simulink model "c221127_FCEV_SLMP_SQP"  (R2022b)
settings: Solver=FixedStepAuto  StartTime=0.0  StopTime=DrvCycLen  FixedStep=1  RelTol=1e-3
values from neighbouring files (symbols this model uses):
  AccThrshd = 1    [Config_c221112.m]    (also in Config_c221127.m; Config_c221218.m; Config_c230117.m; Config_c230321.m)
  AlphaRampFactor = 8    [Config_c221112.m]    (also in Config_c221127.m; Config_c221218.m; Config_c230117.m; Config_c230321.m)
  Bat_eff_chg_average = 0.969    [FCEV_original_data.mat]
  Bat_eff_dis_average = 0.9632    [FCEV_original_data.mat]
  Bat_end_of_life_percent = 20    [FCEV_original_data.mat]
  Bat_I_chg_max = -120    [FCEV_original_data.mat]
  Bat_I_dis_max = 200    [FCEV_original_data.mat]
  Bat_nom_Ic = 2.5    [FCEV_original_data.mat]
  Bat_nom_SOC = 0.35    [FCEV_original_data.mat]
  Bat_nom_temp_oC = 25    [FCEV_original_data.mat]
  Bat_num_pa = 9    [FCEV_original_data.mat]
  Bat_num_se = 97    [FCEV_original_data.mat]
  Bat_ori_C1_chg_F = [397.526659684 455.660832136 435.08783522 460.845064365 457.605812374 417.289828504 416.373906992 359.741413056 321.561704819 1109.14132554 1165.67733205 1135.97600211 ... (72 elements, 9x8)]    [FCEV_original_data.mat]
  Bat_ori_C1_dis_F = [187.121968588 287.083505726 346.448009002 395.529439835 387.517274826 389.973134196 432.856765051 486.92921923 512.158935268 425.990733989 614.68708868 771.472592368 ... (72 elements, 9x8)]    [FCEV_original_data.mat]
  Bat_ori_C2_chg_F = [8748.48589695 7773.35875681 9404.86567646 8934.73981058 8290.58671366 7592.78422269 7759.44623103 7396.59043829 6151.35152293 16187.7227039 11721.8480541 13157.8579836 ... (72 elements, 9x8)]    [FCEV_original_data.mat]
  Bat_ori_C2_dis_F = [2939.81325553 4590.73311898 5504.93546413 5887.5077374 6534.37836712 7765.46899768 10584.7751706 10372.0508438 9238.72693885 5207.86390693 7911.43744944 8879.62137571 ... (72 elements, 9x8)]    [FCEV_original_data.mat]
  Bat_ori_cap_max_Ah = 20.7    [Config_c221218.m]    (also in Config_c230117.m; Config_c230321.m; FCEV_original_data.mat)
  Bat_ori_dUdt4 = [-0.303773584906 -0.249056603774 -0.115094339623 -0.0396226415094 0.0396226415094 0.0641509433962 0.107547169811 0.111320754717 0.0415094339623 0.0547169811321 0.130188679245]    [FCEV_original_data.mat]
  Bat_ori_R0_chg_O = [0.0771669453735 0.0731809311402 0.0726556782939 0.0729965156794 0.0731758310684 0.0742031005051 0.0721266921026 0.0714211058078 0.0714186176143 0.0374124505155 0.0354566732504 0.0345430657188 ... (72 elements, 9x8)]    [FCEV_original_data.mat]
  Bat_ori_R0_dis_O = [0.0819458671157 0.0812429476608 0.0803749674507 0.0805513601722 0.0838629023857 0.0850797840015 0.0829875518672 0.0826388888889 0.0812514106148 0.0428124986417 0.0424658903711 0.0428572670451 ... (72 elements, 9x8)]    [FCEV_original_data.mat]
  Bat_ori_R1_chg_O = [0.114339870884 0.105392753268 0.104421193553 0.109821896183 0.114868279838 0.123333154908 0.129174812826 0.149917249373 0.174896487845 0.0420560161846 0.0390948352938 0.0370122837364 ... (72 elements, 9x8)]    [FCEV_original_data.mat]
  Bat_ori_R1_dis_O = [0.304806399643 0.213604089624 0.171463520004 0.151183840498 0.140630862434 0.128795299077 0.116857791733 0.112567113582 0.106368362501 0.0943235089866 0.0730697254134 0.0611414736086 ... (72 elements, 9x8)]    [FCEV_original_data.mat]
  Bat_ori_R2_chg_O = [0.134518959939 0.17565045702 0.161100627268 0.189032232545 0.205639040497 0.226170473035 0.223651875822 0.181765694192 0.212966950836 0.073628872144 0.0788540822416 0.0792414571734 ... (72 elements, 9x8)]    [FCEV_original_data.mat]
  Bat_ori_R2_dis_O = [0.354968099904 0.285293035102 0.286338708953 0.298763853987 0.248762838155 0.178586175471 0.129047399775 0.188406991173 0.174494800676 0.131839238891 0.123225430215 0.132069033134 ... (72 elements, 9x8)]    [FCEV_original_data.mat]
  Bat_ori_SOC2 = [0 0.001 0.002 0.003 0.004 0.005 0.006 0.007 0.008 0.009 0.01 0.011 ... (1001 elements, 1x1001)]    [FCEV_original_data.mat]
  Bat_ori_SOC4 = [-0.00598301069999 0.0920117618231 0.190864167279 0.289083557951 0.387343788287 0.485011843502 0.5850485992 0.678163031937 0.774810095565 0.876684636119 0.972739524626]    [FCEV_original_data.mat]
  Bat_ori_Uoc_chg_V = [2.4478 2.54923264342 2.6007 2.6383 2.66953057366 2.69636321708 2.7197 2.74042850391 2.75906114733 2.77619379074 2.792 2.80675907757 ... (1001 elements, 1x1001)]    [FCEV_original_data.mat]
  Bat_ori_Uoc_dis_V = [1.9998 2.03916768329 2.24724374236 2.39700902919 2.48767431602 2.5476 2.5882 2.6202 2.64771773167 2.6719 2.6933 2.71251566192 ... (1001 elements, 1x1001)]    [FCEV_original_data.mat]
  Bat_ori_Uoc_V = [2.2238 2.29420016335 2.42397187118 2.5176545146 2.57860244484 2.62198160854 2.65395 2.68031425195 2.7033894395 2.72404689537 2.74265 2.75963736975 ... (1001 elements, 1x1001)]    [FCEV_original_data.mat]
  Bat_power_max_kW = 50    [FCEV_original_data.mat]
  Bat_power_min_kW = 0    [FCEV_original_data.mat]
  Bat_single_capacity_nom_Ah = 2.3    [FCEV_original_data.mat]
  Bat_SOC_ini = 0.3    [Config_c22100601.m]    (also in Config_c22100701.m; FCEV_original_data.mat = 0.45)
  Bat_SOC_max = 0.9    [FCEV_original_data.mat]
  Bat_SOC_min = 0.3    [FCEV_original_data.mat]
  Bat_temp_amb_oC = 25    [FCEV_original_data.mat]
  Bat_temp_cool_oC = 25    [FCEV_original_data.mat]
  BattInitTemp = 25    [Config_c221127.m]    (also in Config_c221218.m; Config_c230117.m; Config_c230321.m)
  BattOnly = 0    [Config_c221218.m]    (also in Config_c230117.m = BattSocRightNow > BattSocLowerLimit; Config_c230321.m = double(BattSocRightNow > BattSocLowerLimit))
  BattSocInit = 0.9    [Config_c221112.m]    (also in Config_c221127.m = 0.3; Config_c221218.m = 0.3; Config_c230117.m = 0.8; Config_c230321.m = 0.8)
  BattSocLowerLimit = 0.25    [Config_c221112.m]    (also in Config_c221127.m = 0.3; Config_c221218.m = 0.3; Config_c230117.m = 0.3; Config_c230321.m = 0.3)
  BattSocRightNow = BattSocRightNow - SocDrop    [Config_c221218.m]    (also in Config_c230117.m; Config_c230321.m)
  BattSocUpperLimit = 0.9    [Config_c221112.m]    (also in Config_c221127.m = 0.8; Config_c221218.m = 0.8; Config_c230117.m = 0.8; Config_c230321.m = 0.8)
  CFWF = 0.5    [Config_c221127.m]    (also in Config_c221218.m; Config_c230117.m; Config_c230321.m)
  DCAC_eff = 0.95    [FCEV_original_data.mat]
  DCDC_ori_eff = [0.95 0.96 0.97 0.976 0.98 0.978 0.973 0.962]    [FCEV_original_data.mat]
  DCDC_ori_power_kW = [0 10 20 30 40 50 60 70]    [FCEV_original_data.mat]
  DeAccThrshd = -1    [Config_c221112.m]    (also in Config_c221127.m; Config_c221218.m; Config_c230117.m; Config_c230321.m)
  DeltaFcPwrRcm_down = 0.5    [Config_c221127.m]    (also in Config_c221218.m; Config_c230117.m; Config_c230321.m)
  DeltaFcPwrRcm_up = 2    [Config_c221127.m]    (also in Config_c221218.m = 3; Config_c230117.m = 4; Config_c230321.m = 4)
  DrvCycRange = sum(DrvCycVps(:,2))    [Config_c221112.m]    (also in Config_c221127.m; Config_c221218.m; Config_c230117.m; Config_c230321.m)
  FC_ori_eff = [0.1 0.33 0.492 0.533 0.559 0.596 0.591 0.562 0.508]    [FCEV_original_data.mat]
  FC_ori_fuel_rate_gps = [0 0.0505050505051 0.0846883468835 0.117260787992 0.149075730471 0.279642058166 0.423011844332 0.593119810202 0.820209973753]    [FCEV_original_data.mat]
  FC_ori_power_kW = [0 2 5 7.5 10 20 30 40 50]    [FCEV_original_data.mat]
  FC_power_max_kW = 50    [FCEV_original_data.mat]
  FC_power_min_kW = 0    [FCEV_original_data.mat]
  FcPwrDropCall = 6    [Config_c221127.m]    (also in Config_c221218.m; Config_c230117.m; Config_c230321.m)
  HydpriceRmb = 30    [Config_c221127.m]    (also in Config_c221218.m; Config_c230117.m; Config_c230321.m)
  m = Time_sample    [Config_c22100601.m]    (also in Config_c22100701.m)
  MC_eff_brk_average = 0.810578512397    [FCEV_original_data.mat]
  MC_eff_dri_average = 0.810578512397    [FCEV_original_data.mat]
  MC_inertia = 0.06    [FCEV_original_data.mat]
  MC_ori_eff = [0.7 0.78 0.85 0.86 0.81 0.82 0.79 0.78 0.78 0.78 0.78 0.7 ... (231 elements, 11x21)]    [FCEV_original_data.mat]
  MC_ori_power_brk_req_kW = [0 -28.3912930389 -56.7825860779 -85.1738791168 -113.565172156 -141.956465195 -170.347758234 -198.739051273 -227.130344311 -255.52163735 -283.912930389 0 ... (121 elements, 11x11)]    [FCEV_original_data.mat]
  MC_ori_power_dri_req_kW = [0 0 0 0 0 0 0 0 0 0 0 0 ... (121 elements, 11x11)]    [FCEV_original_data.mat]
  MC_ori_spd_rpm = [0 1000 2000 3000 4000 5000 6000 7000 8000 9000 10000]    [FCEV_original_data.mat]
  MC_ori_trq_brk_max_Nm = [-271.1368 -271.1368 -271.1368 -237.5159 -178.1369 -142.4824 -118.7579 -101.8119 -89.0685 -79.172 -71.1734]    [FCEV_original_data.mat]
  MC_ori_trq_brk_Nm = [-271.136848522 -244.02316367 -216.909478817 -189.795793965 -162.682109113 -135.568424261 -108.454739409 -81.3410545565 -54.2273697044 -27.1136848522 0]    [FCEV_original_data.mat]
  MC_ori_trq_dri_max_Nm = [271.1368 271.1368 271.1368 237.5159 178.1369 142.4824 118.7579 101.8119 89.0685 79.172 71.1734]    [FCEV_original_data.mat]
  MC_ori_trq_dri_Nm = [0 27.1136848522 54.2273697044 81.3410545565 108.454739409 135.568424261 162.682109113 189.795793965 216.909478817 244.02316367 271.136848522]    [FCEV_original_data.mat]
  MC_ori_trq_Nm = [-271.136848522 -244.02316367 -216.909478817 -189.795793965 -162.682109113 -135.568424261 -108.454739409 -81.3410545565 -54.2273697044 -27.1136848522 0 27.1136848522 ... (21 elements, 1x21)]    [FCEV_original_data.mat]
  MC_power_max_kW = 75    [FCEV_original_data.mat]
  MC_spd_max_rpm = 10000    [FCEV_original_data.mat]
  MC_spd_min_rpm = 0    [FCEV_original_data.mat]
  MC_spd_scale = 1    [FCEV_original_data.mat]
  MC_trq_scale = 1    [FCEV_original_data.mat]
  MC_U_min_V = 120    [FCEV_original_data.mat]
  no_FcPwrSlowDrop = 1    [Config_c230321.m]
  Placeholder = 0    [Config_c221127.m]    (also in Config_c221218.m; Config_c230117.m; Config_c230321.m)
  PredLen = 5    [Config_c221112.m]    (also in Config_c221127.m; Config_c221218.m; Config_c230117.m; Config_c230321.m)
  Road_u = 0.75    [FCEV_original_data.mat]
  SC_np = 1    [Config_c230321.m]
  SC_ns = 100    [Config_c230321.m]
  SC_rc = 1000    [Config_c230321.m]
  SLMP_LearningRate = 0.05    [Config_c221112.m]    (also in Config_c221127.m; Config_c221218.m; Config_c230117.m; Config_c230321.m)
  tDegTable = [zeros(1,3),linspace(0,0.13,47)]    [Config_c221127.m]    (also in Config_c221218.m; Config_c230117.m; Config_c230321.m)
  usd2rmb = 7.116    [Config_c22100601.m]    (also in Config_c22100701.m; Config_c221106.m = 6; Config_c221112.m = 6; Config_c221127.m = 6)
  Veh_air_density_kgpm2 = 1.2    [FCEV_original_data.mat]
  Veh_brk_front = [1 0.6 0.608 0.61 0.618 0.624 0.636 0.645 0.655]    [FCEV_original_data.mat]
  Veh_brk_z = [0.1 0.2 0.3 0.4 0.5 0.6 0.7 0.8 0.9]    [FCEV_original_data.mat]
  Veh_brk_z_max = 0.7    [FCEV_original_data.mat]
  Veh_brk_z_min = 0.1    [FCEV_original_data.mat]
  Veh_coeff_drag = 0.312    [FCEV_original_data.mat]
  Veh_coeff_roll = 0.00863    [FCEV_original_data.mat]
  Veh_final_drive_inertia = 0.1105    [FCEV_original_data.mat]
  Veh_final_drive_ratio = 3.47    [FCEV_original_data.mat]
  Veh_frontal_area_m2 = 2.06    [FCEV_original_data.mat]
  Veh_gravity_acc_ms2 = 9.81    [FCEV_original_data.mat]
  Veh_mass_cargo_kg = 113    [FCEV_original_data.mat]
  Veh_mass_curb_kg = 1157    [FCEV_original_data.mat]
  Veh_mech_eff = 0.9    [FCEV_original_data.mat]
  Veh_rotary_mass_conversion_factor = 1.05    [FCEV_original_data.mat]
  Veh_size_cg_height_m = 0.53    [FCEV_original_data.mat]
  Veh_wheel_inertia = 3.1039    [FCEV_original_data.mat]
  Veh_wheel_radius_m = 0.313    [FCEV_original_data.mat]
  Veh_wt_frac_front = 0.5    [FCEV_original_data.mat]
  VstdThrshd = 2    [Config_c221112.m]    (also in Config_c221127.m; Config_c221218.m; Config_c230117.m; Config_c230321.m)
undefined symbols (not defined in the file or in its folder): Bat_ori_temp, SC_iv, SC_nm, SC_SocTable
libraries: autolibshared x2
(part 2 of 8)

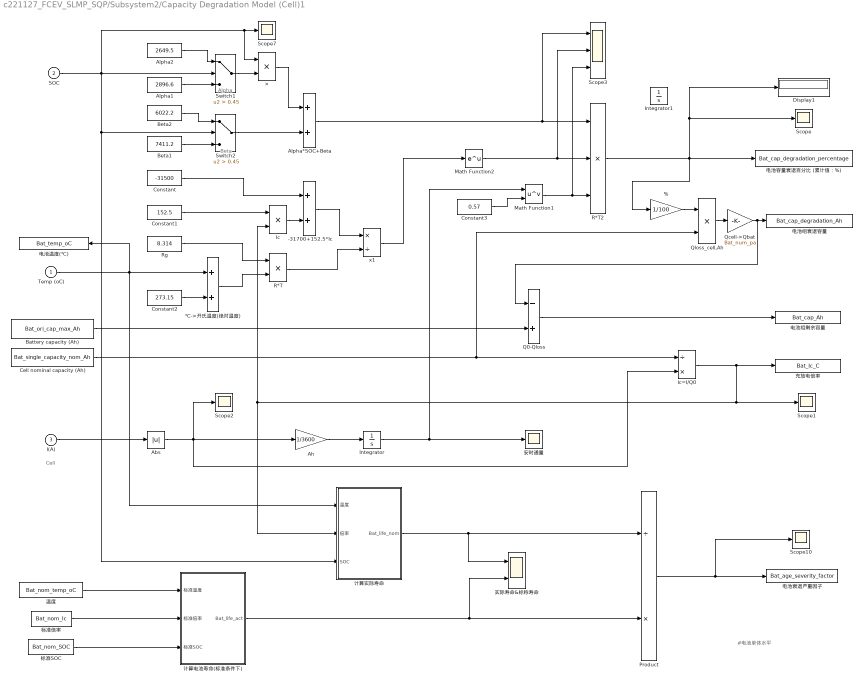
== system c221127_FCEV_SLMP_SQP/Subsystem2/Capacity Degradation Model (Cell)1 ==
  note: Cell
  note: #电池单体水平
  note: Beta
  note: Alpha
  Temp (oC) : Inport
  SOC : Inport  Port=2
  I(A) : Inport  Port=3
  % : Gain  Gain=1/100
  -31700+152.5*Ic : Sum  InputSameDT=on  SaturateOnIntegerOverflow=on  OutDataTypeStr=Inherit: Same as first input
  Abs : Abs  SaturateOnIntegerOverflow=off
  Ah : Gain  Gain=1/3600
  Alpha*SOC+Beta : Sum  InputSameDT=on  SaturateOnIntegerOverflow=on  OutDataTypeStr=Inherit: Same as first input
  Alpha1 : Constant  Value=2896.6
  Alpha2 : Constant  Value=2649.5
  Battery capacity (Ah) : Constant  Value=Bat_ori_cap_max_Ah
  Beta1 : Constant  Value=7411.2
  Beta2 : Constant  Value=6022.2
  Cell nominal capacity (Ah) : Constant  Value=Bat_single_capacity_nom_Ah
  Constant : Constant  Value=-31500
  Constant1 : Constant  Value=152.5
  Constant2 : Constant  Value=273.15
  Constant3 : Constant  Value=0.57
  Display1 : Display
  Ic : Product  InputSameDT=on  RndMeth=Zero  SaturateOnIntegerOverflow=on  OutDataTypeStr=Inherit: Same as first input
  Ic=I/Q0 : Product  Inputs=/*  InputSameDT=on  RndMeth=Zero  SaturateOnIntegerOverflow=on  OutDataTypeStr=Inherit: Same as first input
  Integrator : Integrator  InitialCondition=eps
  Integrator1 : Integrator
  Math Function1 : Math  Operator=pow  SignedPower=on
  Math Function2 : Math  SignedPower=on
  Product : Product  Inputs=/*
  Q0-Qloss : Sum  Inputs=-+  InputSameDT=on  SaturateOnIntegerOverflow=on  OutDataTypeStr=Inherit: Same as first input
  Qcell->Qbat : Gain  Gain=Bat_num_pa  SaturateOnIntegerOverflow=on  OutDataTypeStr=Inherit: Same as input  ParamDataTypeStr=Inherit: Same as input
  Qloss_cell,Ah : Product  InputSameDT=on  RndMeth=Zero  SaturateOnIntegerOverflow=on  OutDataTypeStr=Inherit: Same as first input
  R*T : Product  InputSameDT=on  RndMeth=Zero  SaturateOnIntegerOverflow=on  OutDataTypeStr=Inherit: Same as first input
  R*T2 : Product  Inputs=3  InputSameDT=on  RndMeth=Zero  SaturateOnIntegerOverflow=on  OutDataTypeStr=Inherit: Same as first input
  Rg : Constant  Value=8.314
  Scope{,1..2,7,10} (5 alike) : Scope
  Scope3 : Scope  NumInputPorts=3
  Switch1 : Switch  Criteria=u2 > Threshold  Threshold=0.45
  Switch2 : Switch  Criteria=u2 > Threshold  Threshold=0.45
  x1 : Product  Inputs=*/  InputSameDT=on  RndMeth=Zero  SaturateOnIntegerOverflow=on  OutDataTypeStr=Inherit: Same as first input
  × : Product  InputSameDT=on  RndMeth=Zero  SaturateOnIntegerOverflow=on  OutDataTypeStr=Inherit: Same as first input
  ℃->开氏温度(绝对温度) : Sum  InputSameDT=on  SaturateOnIntegerOverflow=on  OutDataTypeStr=Inherit: Same as first input
  充放电倍率 : ToWorkspace  VariableName=Bat_Ic_C  SampleTime=-1
  安时通量 : Scope
  实际寿命&标称寿命 : Scope  NumInputPorts=2
  标准SOC : Constant  Value=Bat_nom_SOC
  标准倍率 : Constant  Value=Bat_nom_Ic
  温度 : Constant  Value=Bat_nom_temp_oC  VectorParams1D=off
  电池容量衰退百分比 (累计值：%) : ToWorkspace  VariableName=Bat_cap_degradation_percentage  SampleTime=-1
  电池温度(℃) : ToWorkspace  VariableName=Bat_temp_oC  SampleTime=-1
  电池组剩余容量 : ToWorkspace  VariableName=Bat_cap_Ah  SampleTime=-1
  电池组衰退容量 : ToWorkspace  VariableName=Bat_cap_degradation_Ah  SampleTime=-1
  电池衰退严重因子 : ToWorkspace  VariableName=Bat_age_severity_factor  SampleTime=-1
  计算实际寿命 : Subsystem
  计算电池寿命(标准条件下) : Subsystem
  wires:
  SOC/1 -> Switch1/2, Scope7/1, ×/1, Switch2/2, 计算实际寿命/3(SOC)
  Alpha2/1 -> Switch1/1
  Alpha1/1 -> Switch1/3
  Beta2/1 -> Switch2/1
  Beta1/1 -> Switch2/3
  Switch1/1 -> ×/2
  Switch2/1 -> Alpha*SOC+Beta/2
  ×/1 -> Alpha*SOC+Beta/1
  Rg/1 -> R*T/1
  ℃->开氏温度(绝对温度)/1 -> R*T/2
  Ic=I/Q0/1 -> Scope1/1, Ic/2, 计算实际寿命/2(倍率), 充放电倍率/1
  Alpha*SOC+Beta/1 -> R*T2/1, Scope3/1
  Constant/1 -> -31700+152.5*Ic/1
  Ic/1 -> -31700+152.5*Ic/2
  Constant1/1 -> Ic/1
  -31700+152.5*Ic/1 -> x1/1
  R*T/1 -> x1/2
  Math Function2/1 -> R*T2/2, Scope3/2
  x1/1 -> Math Function2/1
  Math Function1/1 -> R*T2/3, Scope3/3
  R*T2/1 -> Scope/1, Display1/1, 电池容量衰退百分比 (累计值：%)/1, %/1
  Abs/1 -> Ic=I/Q0/2, Ah/1, Scope2/1
  Integrator/1 -> Math Function1/1, 安时通量/1
  Temp (oC)/1 -> 计算实际寿命/1(温度), 电池温度(℃)/1, ℃->开氏温度(绝对温度)/1
  Constant2/1 -> ℃->开氏温度(绝对温度)/2
  %/1 -> Qloss_cell,Ah/1
  温度/1 -> 计算电池寿命(标准条件下)/1(标准温度)
  标准倍率/1 -> 计算电池寿命(标准条件下)/2(标准倍率)
  标准SOC/1 -> 计算电池寿命(标准条件下)/3(标准SOC)
  Product/1 -> 电池衰退严重因子/1, Scope10/1
  计算实际寿命/1(Bat_life_nom) -> 实际寿命&标称寿命/1, Product/1
  计算电池寿命(标准条件下)/1(Bat_life_act) -> Product/2, 实际寿命&标称寿命/2
  I(A)/1 -> Abs/1
  Cell nominal capacity (Ah)/1 -> Qloss_cell,Ah/2, Ic=I/Q0/1
  Qcell->Qbat/1 -> Q0-Qloss/1, 电池组衰退容量/1
  Qloss_cell,Ah/1 -> Qcell->Qbat/1
  Battery capacity (Ah)/1 -> Q0-Qloss/2
  Q0-Qloss/1 -> 电池组剩余容量/1
  Ah/1 -> Integrator/1
  Constant3/1 -> Math Function1/2

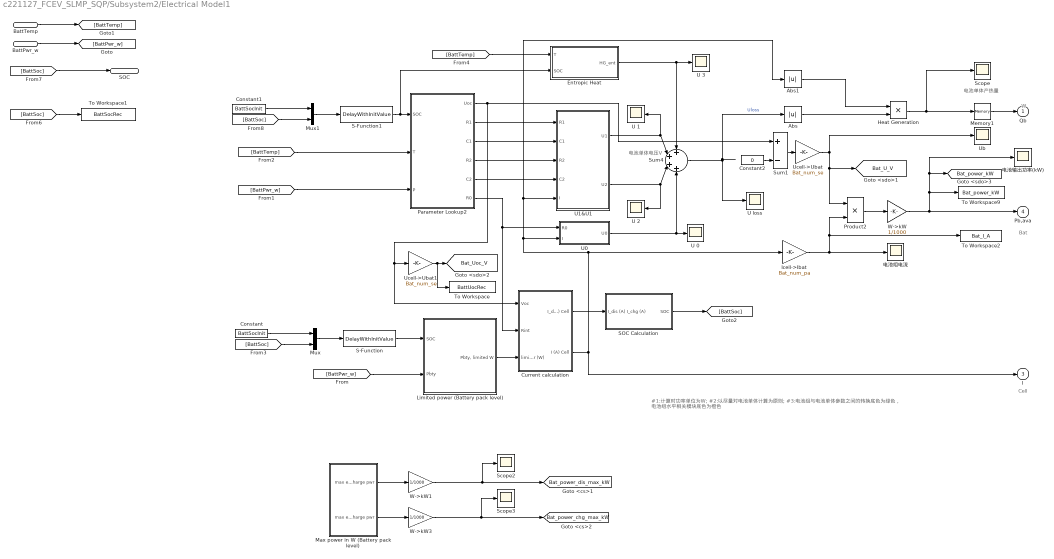
== system c221127_FCEV_SLMP_SQP/Subsystem2/Electrical Model1 ==
  note: Bat
  note: Cell
  note: #1:计算时功率单位为W;
      | #2:以尽量对电池单体计算为原则;
      | #3:电池组与电池单体参数之间的转换底色为绿色， 电池组水平相关模块底色为橙色
  note: W
  note: 电池单体产热量
  note: 电池单体电压V
  BattTemp : Inport
  BattPwr_w : Inport  Port=2
  Abs : Abs  SaturateOnIntegerOverflow=off
  Abs1 : Abs  SaturateOnIntegerOverflow=off
  Constant : Constant  Value=BattSocInit
  Constant1 : Constant  Value=BattSocInit
  Constant2 : Constant  Value=0
  Current calculation : Subsystem
  Entropic Heat : Subsystem
  Heat Generation : Product  RndMeth=Zero
  Icell->Ibat : Gain  Gain=Bat_num_pa  SaturateOnIntegerOverflow=on  OutDataTypeStr=Inherit: Same as input  ParamDataTypeStr=Inherit: Same as input
  Limited power (Battery pack level) : Subsystem
  Max power in W (Battery pack level) : Subsystem
  Memory1 : Memory  InheritSampleTime=on
  Mux : Mux  Inputs=2
  Mux1 : Mux  Inputs=2
  Parameter Lookup2 : Subsystem
  Product2 : Product  RndMeth=Zero
  S-Function : S-Function  FunctionName=DelayWithInitValue  SFunctionDeploymentMode=off  EnableBusSupport=off
  S-Function1 : S-Function  FunctionName=DelayWithInitValue  SFunctionDeploymentMode=off  EnableBusSupport=off
  SOC Calculation : Subsystem
  Scope : Scope
  Scope2 : Scope
  Scope3 : Scope
  Sum1 : Sum  Inputs=+-
  Sum4 : Sum  Inputs=++++
  To Workspace : ToWorkspace  VariableName=BattUocRec  SaveFormat=Timeseries  SampleTime=-1
  To Workspace1 : ToWorkspace  VariableName=BattSocRec  SampleTime=-1
  To Workspace2 : ToWorkspace  VariableName=Bat_I_A  SampleTime=-1
  To Workspace9 : ToWorkspace  VariableName=Bat_power_kW  SampleTime=-1
  U {0..3} (4 alike) : Scope
  U loss : Scope
  U0 : Subsystem
  U1&U1 : Subsystem
  Ub : Scope
  Ucell->Ubat : Gain  Gain=Bat_num_se  SaturateOnIntegerOverflow=on  OutDataTypeStr=Inherit: Same as input  ParamDataTypeStr=Inherit: Same as input
  Ucell->Ubat1 : Gain  Gain=Bat_num_se  SaturateOnIntegerOverflow=on  OutDataTypeStr=Inherit: Same as input  ParamDataTypeStr=Inherit: Same as input
  W->kW : Gain  Gain=1/1000  SaturateOnIntegerOverflow=on  OutDataTypeStr=Inherit: Same as input  ParamDataTypeStr=Inherit: Same as input
  W->kW1 : Gain  Gain=1/1000  SaturateOnIntegerOverflow=on  OutDataTypeStr=Inherit: Same as input  ParamDataTypeStr=Inherit: Same as input
  W->kW3 : Gain  Gain=1/1000  SaturateOnIntegerOverflow=on  OutDataTypeStr=Inherit: Same as input  ParamDataTypeStr=Inherit: Same as input
  电池组电流 : Scope
  电池输出功率(kW) : Scope
  Qb : Outport  InitialOutput=0
  SOC : Outport  Port=2  InitialOutput=0
  I : Outport  Port=3  InitialOutput=0
  Pb,ava : Outport  Port=4  InitialOutput=0
  tag scope: Bat_U_V=global, Bat_Uoc_V=global, Bat_power_chg_max_kW=global, Bat_power_dis_max_kW=global, Bat_power_kW=global
  wires:
  Parameter Lookup2/2(R1) -> U1&U1/1(R1)
  Parameter Lookup2/3(C1) -> U1&U1/2(C1)
  Parameter Lookup2/4(R2) -> U1&U1/3(R2)
  Parameter Lookup2/5(C2) -> U1&U1/4(C2)
  Parameter Lookup2/6(R0) -> U0/1(R0), Current calculation/2(Rint)
  U1&U1/1(U1) -> Sum4/2, U 1/1
  U1&U1/2(U2) -> U 2/1, Sum4/3
  Ucell->Ubat/1 -> Product2/1, [Bat_U_V], Ub/1
  Entropic Heat/1(HG_ent) -> U 3/1, Sum4/1
  Product2/1 -> W->kW/1
  W->kW/1 -> 电池输出功率(kW)/1, [Bat_power_kW], To Workspace9/1, Pb,ava/1
  Memory1/1 -> Qb/1
  Heat Generation/1 -> Scope/1, Memory1/1
  Current calculation/1(I_dis (A) I_chg (A) Cell) -> SOC Calculation/1(I_dis (A) I_chg (A))
  [BattTemp] -> Parameter Lookup2/2(T)
  [BattPwr_w] -> Limited power (Battery pack level)/2(Pbty)
  Icell->Ibat/1 -> Product2/2, To Workspace2/1, 电池组电流/1
  W->kW1/1 -> Scope2/1, [Bat_power_dis_max_kW]
  W->kW3/1 -> Scope3/1, [Bat_power_chg_max_kW]
  Max power in W (Battery pack level)/1(max ess discharge pwr) -> W->kW1/1
  Max power in W (Battery pack level)/2(max ess charge pwr) -> W->kW3/1
  Parameter Lookup2/1(Uoc) -> Sum1/1, Ucell->Ubat1/1, Current calculation/1(Voc)
  Ucell->Ubat1/1 -> To Workspace/1, [Bat_Uoc_V]
  Limited power (Battery pack level)/1("Pbty, limited W") -> Current calculation/3(limited output power (W))
  Current calculation/2(I (A) Cell) -> Abs1/1, U1&U1/5(I), U0/2(I), Icell->Ibat/1, I/1
  U0/1(U0) -> U 0/1, Sum4/4
  Sum4/1 -> Abs/1, U loss/1  "Uloss"
  Sum1/1 -> Ucell->Ubat/1
  Abs/1 -> Heat Generation/2
  Abs1/1 -> Heat Generation/1
  BattPwr_w/1 -> [BattPwr_w]
  [BattPwr_w] -> Parameter Lookup2/3(P)
  BattTemp/1 -> [BattTemp]
  Mux/1 -> S-Function/1
  Constant/1 -> Mux/1
  [BattSoc] -> Mux/2
  S-Function/1 -> Limited power (Battery pack level)/1(SOC)
  SOC Calculation/1(SOC) -> [BattSoc]
  S-Function1/1 -> Entropic Heat/2(SOC), Parameter Lookup2/1(SOC)
  [BattSoc] -> To Workspace1/1
  [BattSoc] -> SOC/1
  [BattSoc] -> Mux1/2
  Constant1/1 -> Mux1/1
  Mux1/1 -> S-Function1/1
  [BattTemp] -> Entropic Heat/1(T)
  Constant2/1 -> Sum1/2

== system c221127_FCEV_SLMP_SQP/Subsystem2/Thermal Model1 ==
  note: 需要设置温度初始值
  note: W
  note: Tf
  note: (k)
  note: 冷却液温度 ℃
  note: ℃
  note: ℃
  Qb : Inport
  (1-1/RsCs-1/RcCs)*Ts(k-1) : Product  Inputs=**  RndMeth=Zero
  (RC*Cc-1)*Tc(k-1)/RcCc : Product  Inputs=**  RndMeth=Zero
  (RC*Cc-1)/RcCc : Product  Inputs=*/  RndMeth=Zero
  Calculation : Subsystem
  Constant : Constant  Value=273
  Constant3 : Constant
  Math Function : Math  Operator=reciprocal  SignedPower=on
  Math Function1 : Math  Operator=reciprocal  SignedPower=on
  Qb(k-1)/Cc : Product  Inputs=*/  RndMeth=Zero
  Sum10 : Sum  Inputs=+++
  Sum11 : Sum  Inputs=+--|
  Sum3 : Sum  Inputs=+++
  Sum4 : Sum  Inputs=+-|
  Sum5 : Sum  Inputs=|+-
  Sum7 : Sum  Inputs=++|
  Sum9 : Sum  Inputs=-+|
  Tc (K) : Scope
  Tc (℃) : Scope
  Tc(k-1) : Memory  InitialCondition=Bat_temp_amb_oC+273.15  InheritSampleTime=on
  Tc(k-1)/RcCs : Product  Inputs=*/  RndMeth=Zero
  Tf/RsCs : Product  Inputs=*/  RndMeth=Zero
  Tf1 : Constant  Value=Bat_temp_cool_oC
  Ts (K) : Scope
  Ts (℃) : Scope
  Ts(k-1) : Memory  InitialCondition=Bat_temp_amb_oC+273.15  InheritSampleTime=on
  Ts(k-1)/RcCc : Product  Inputs=*/  RndMeth=Zero
  Tc. : Outport
  Ts. : Outport  Port=2
  wires:
  Calculation/1(Cc) -> Qb(k-1)/Cc/2
  Calculation/2(RcCc) -> (RC*Cc-1)/RcCc/2, Ts(k-1)/RcCc/2, Sum4/1
  Constant3/1 -> Sum11/1, Sum4/2
  Sum4/1 -> (RC*Cc-1)/RcCc/1
  Qb(k-1)/Cc/1 -> Sum3/1
  Ts(k-1)/RcCc/1 -> Sum3/2
  Tf1/1 -> Sum7/2
  Calculation/3(RsCs) -> Tf/RsCs/2, Math Function/1
  Sum7/1 -> Tf/RsCs/1
  Tf/RsCs/1 -> Sum10/1
  Calculation/4(RcCs) -> Tc(k-1)/RcCs/2, Math Function1/1
  Math Function1/1 -> Sum11/2
  Math Function/1 -> Sum11/3
  (1-1/RsCs-1/RcCs)*Ts(k-1)/1 -> Sum10/2
  Sum11/1 -> (1-1/RsCs-1/RcCs)*Ts(k-1)/1
  Tc(k-1)/RcCs/1 -> Sum10/3
  Sum3/1 -> Sum5/1, Tc(k-1)/1, Tc (K)/1
  Constant/1 -> Sum9/1, Sum5/2, Sum7/1
  Sum5/1 -> Tc (℃)/1, Tc./1
  Sum10/1 -> Sum9/2, Ts(k-1)/1, Ts (K)/1
  Sum9/1 -> Ts./1, Ts (℃)/1
  Ts(k-1)/1 -> Ts(k-1)/RcCc/1, (1-1/RsCs-1/RcCs)*Ts(k-1)/2
  (RC*Cc-1)*Tc(k-1)/RcCc/1 -> Sum3/3
  (RC*Cc-1)/RcCc/1 -> (RC*Cc-1)*Tc(k-1)/RcCc/1
  Tc(k-1)/1 -> Tc(k-1)/RcCs/1, (RC*Cc-1)*Tc(k-1)/RcCc/2
  Qb/1 -> Qb(k-1)/Cc/1

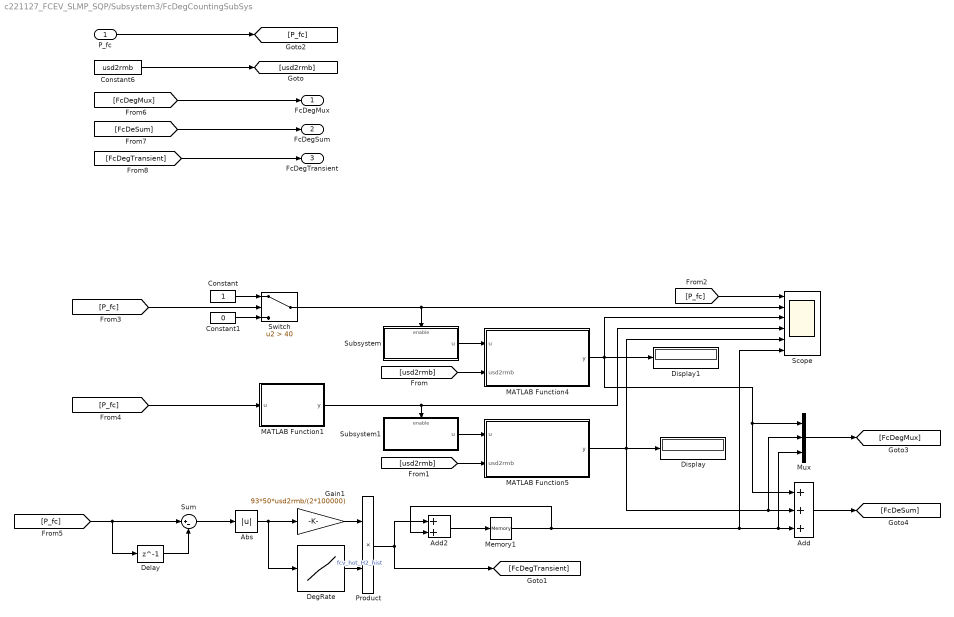
== system c221127_FCEV_SLMP_SQP/Subsystem3/FcDegCountingSubSys ==
  P_fc : Inport
  Abs : Abs  SaturateOnIntegerOverflow=off
  Add : Sum  Inputs=+++
  Add2 : Sum
  Constant : Constant
  Constant1 : Constant  Value=0
  Constant6 : Constant  Value=usd2rmb
  DegRate : Lookup_n-D  NumberOfTableDimensions=1  BreakpointsForDimension1=1:50  Table=tDegTable  RndMeth=Simplest
  Delay : Delay  DelayLength=1
  Display : Display
  Display1 : Display
  Gain1 : Gain  Gain=93*50*usd2rmb/(2*100000)
  MATLAB Function1 : MATLAB Function  TreatAsAtomicUnit=on
  MATLAB Function4 : MATLAB Function  TreatAsAtomicUnit=on
  MATLAB Function5 : MATLAB Function  TreatAsAtomicUnit=on
  Memory1 : Memory
  Mux : Mux  Inputs=3
  Product : Product
  Scope : Scope  NumInputPorts=6
  Subsystem : Subsystem
  Subsystem1 : Subsystem
  Sum : Sum  Inputs=|+-
  Switch : Switch  Criteria=u2 > Threshold  Threshold=40  SaturateOnIntegerOverflow=off  InputSameDT=off
  FcDegMux : Outport
  FcDegSum : Outport  Port=2
  FcDegTransient : Outport  Port=3
  wires:
  MATLAB Function5/1(y) -> Scope/5, Display/1, Mux/2, Add/2
  MATLAB Function1/1(y) -> Subsystem1/Enable, Scope/4
  Subsystem/1(u) -> MATLAB Function4/1(u)
  Constant/1 -> Switch/1
  [usd2rmb] -> MATLAB Function4/2(usd2rmb)
  Constant1/1 -> Switch/3
  [usd2rmb] -> MATLAB Function5/2(usd2rmb)
  Switch/1 -> Scope/2, Subsystem/Enable
  P_fc/1 -> [P_fc]
  Subsystem1/1(u) -> MATLAB Function5/1(u)
  MATLAB Function4/1(y) -> Scope/3, Mux/1, Add/1, Display1/1
  Constant6/1 -> [usd2rmb]
  [P_fc] -> Scope/1
  Memory1/1 -> Scope/6, Mux/3, Add/3, Add2/2
  Add2/1 -> Memory1/1
  Sum/1 -> Abs/1
  Abs/1 -> DegRate/1, Gain1/1
  Delay/1 -> Sum/2
  [P_fc] -> Delay/1, Sum/1
  [P_fc] -> Switch/2
  Add/1 -> [FcDeSum]
  Mux/1 -> [FcDegMux]
  [P_fc] -> MATLAB Function1/1(u)
  [FcDegMux] -> FcDegMux/1
  [FcDeSum] -> FcDegSum/1
  [FcDegTransient] -> FcDegTransient/1
  Product/1 -> [FcDegTransient], Add2/1
  Gain1/1 -> Product/1
  DegRate/1 -> Product/2  "fcv_hot_H2_hist"

== system c221127_FCEV_SLMP_SQP/Subsystem3/Fuel Rate Calculation1 ==
  note: Transient load response
  fc pwr : Inport
  "FC hydrogen consumption rate " : Lookup_n-D  NumberOfTableDimensions=1  BreakpointsForDimension1=FC_ori_power_kW  Table=FC_ori_fuel_rate_gps  RndMeth=Simplest
  fcv_H2_rate (g/s)1 : Outport
  wires:
  fc pwr/1 -> "FC hydrogen consumption rate "/1
  "FC hydrogen consumption rate "/1 -> fcv_H2_rate (g/s)1/1  "fcv_hot_H2_hist"

== system c221127_FCEV_SLMP_SQP/Subsystem3/Fuel cell efficiency calculation ==
  note: Carryover
  note: Transient load response
  fc power : Inport
  "FC efficiency " : Lookup_n-D  NumberOfTableDimensions=1  BreakpointsForDimension1=FC_ori_power_kW  Table=FC_ori_eff  RndMeth=Simplest
  "fc_eff " : Outport
  wires:
  "FC efficiency "/1 -> "fc_eff "/1
  fc power/1 -> "FC efficiency "/1

== system c221127_FCEV_SLMP_SQP/Subsystem3/Power Calculation ==
  note: Transient load response
  fc on : Inport
  Power command (kW) : Inport  Port=2
  "   " : Constant  Value=0
  Switch2 : Switch  Threshold=0.5
  Power output (kW) : Outport
  wires:
  "   "/1 -> Switch2/3
  Power command (kW)/1 -> Switch2/1
  fc on/1 -> Switch2/2
  Switch2/1 -> Power output (kW)/1

== system c221127_FCEV_SLMP_SQP/Subsystem4/VehModel_Pred+1 ==
  note: CarryOver
  Pred_v1 : Inport
  Enable : EnablePort
  Gain : Gain  Gain=3.6
  Power bus : Subsystem
  主减及变速器模型 : Subsystem
  整车动力学模型 : Subsystem
  车轮模型 : Subsystem
  驱动电机模型 : Subsystem
  PredPwr_1 : Outport
  wires:
  主减及变速器模型/1(drive torque (Nm) speed (rad/s) brike torque (Nm) req'd at input side of final drive) -> 驱动电机模型/1(drive torque (Nm) speed (rad/s) brake torque (Nm) req'd at motor)
  驱动电机模型/1(drive power (kW) brake power (kW) req'd motor input power (电功率)) -> Power bus/1(drive power (kW) brake power (kW) req at power bus)
  整车动力学模型/1(需求驱动力N 目标车速m/s 需求制动力N) -> 车轮模型/1("tractive force, brake force and speed req'd of tire/road interface 需求驱动力N 目标车速m/s 需求制动力N")
  车轮模型/1(drive torque (Nm) speed (rad/s) brake torque (Nm) req'd from drivetrain into axle) -> 主减及变速器模型/1(drive torque (Nm) speed (rad/s) brake torque (Nm) req'd at output side of final drive)
  Pred_v1/1 -> Gain/1
  Power bus/1(drive power (kW)/brake power (kW) req from power sources) -> PredPwr_1/1
  Gain/1 -> 整车动力学模型/1(需求车速 km/h)

== system c221127_FCEV_SLMP_SQP/Subsystem4/VehModel_Pred+2 ==
  note: CarryOver
  Pred_v2 : Inport
  Pred_v1 : Inport  Port=2
  Enable : EnablePort
  Gain : Gain  Gain=3.6
  Gain1 : Gain  Gain=3.6
  Power bus : Subsystem
  主减及变速器模型 : Subsystem
  整车动力学模型 : Subsystem
  车轮模型 : Subsystem
  驱动电机模型 : Subsystem
  PredPwr_2 : Outport
  wires:
  主减及变速器模型/1(drive torque (Nm) speed (rad/s) brike torque (Nm) req'd at input side of final drive) -> 驱动电机模型/1(drive torque (Nm) speed (rad/s) brake torque (Nm) req'd at motor)
  驱动电机模型/1(drive power (kW) brake power (kW) req'd motor input power (电功率)) -> Power bus/1(drive power (kW) brake power (kW) req at power bus)
  整车动力学模型/1(需求驱动力N 目标车速m/s 需求制动力N) -> 车轮模型/1("tractive force, brake force and speed req'd of tire/road interface 需求驱动力N 目标车速m/s 需求制动力N")
  车轮模型/1(drive torque (Nm) speed (rad/s) brake torque (Nm) req'd from drivetrain into axle) -> 主减及变速器模型/1(drive torque (Nm) speed (rad/s) brake torque (Nm) req'd at output side of final drive)
  Pred_v2/1 -> Gain/1
  Power bus/1(drive power (kW)/brake power (kW) req from power sources) -> PredPwr_2/1
  Gain/1 -> 整车动力学模型/1(需求车速 km/h)
  Pred_v1/1 -> Gain1/1
  Gain1/1 -> 整车动力学模型/2(Temp)

== system c221127_FCEV_SLMP_SQP/Subsystem4/VehModel_Pred+3 ==
  note: CarryOver
  Pred_v3 : Inport
  Pred_v2 : Inport  Port=2
  Enable : EnablePort
  Gain : Gain  Gain=3.6
  Gain1 : Gain  Gain=3.6
  Power bus : Subsystem
  主减及变速器模型 : Subsystem
  整车动力学模型 : Subsystem
  车轮模型 : Subsystem
  驱动电机模型 : Subsystem
  PredPwr_3 : Outport
  wires:
  主减及变速器模型/1(drive torque (Nm) speed (rad/s) brike torque (Nm) req'd at input side of final drive) -> 驱动电机模型/1(drive torque (Nm) speed (rad/s) brake torque (Nm) req'd at motor)
  驱动电机模型/1(drive power (kW) brake power (kW) req'd motor input power (电功率)) -> Power bus/1(drive power (kW) brake power (kW) req at power bus)
  整车动力学模型/1(需求驱动力N 目标车速m/s 需求制动力N) -> 车轮模型/1("tractive force, brake force and speed req'd of tire/road interface 需求驱动力N 目标车速m/s 需求制动力N")
  车轮模型/1(drive torque (Nm) speed (rad/s) brake torque (Nm) req'd from drivetrain into axle) -> 主减及变速器模型/1(drive torque (Nm) speed (rad/s) brake torque (Nm) req'd at output side of final drive)
  Pred_v3/1 -> Gain/1
  Power bus/1(drive power (kW)/brake power (kW) req from power sources) -> PredPwr_3/1
  Gain/1 -> 整车动力学模型/1(需求车速 km/h)
  Pred_v2/1 -> Gain1/1
  Gain1/1 -> 整车动力学模型/2(需求车速 km/h1)

== system c221127_FCEV_SLMP_SQP/Subsystem4/VehModel_Pred+4 ==
  note: CarryOver
  Pred_v4 : Inport
  Pred_v3 : Inport  Port=2
  Enable : EnablePort
  Gain : Gain  Gain=3.6
  Gain1 : Gain  Gain=3.6
  Power bus : Subsystem
  主减及变速器模型 : Subsystem
  整车动力学模型 : Subsystem
  车轮模型 : Subsystem
  驱动电机模型 : Subsystem
  PredPwr_4 : Outport
  wires:
  主减及变速器模型/1(drive torque (Nm) speed (rad/s) brike torque (Nm) req'd at input side of final drive) -> 驱动电机模型/1(drive torque (Nm) speed (rad/s) brake torque (Nm) req'd at motor)
  驱动电机模型/1(drive power (kW) brake power (kW) req'd motor input power (电功率)) -> Power bus/1(drive power (kW) brake power (kW) req at power bus)
  整车动力学模型/1(需求驱动力N 目标车速m/s 需求制动力N) -> 车轮模型/1("tractive force, brake force and speed req'd of tire/road interface 需求驱动力N 目标车速m/s 需求制动力N")
  车轮模型/1(drive torque (Nm) speed (rad/s) brake torque (Nm) req'd from drivetrain into axle) -> 主减及变速器模型/1(drive torque (Nm) speed (rad/s) brake torque (Nm) req'd at output side of final drive)
  Pred_v4/1 -> Gain/1
  Power bus/1(drive power (kW)/brake power (kW) req from power sources) -> PredPwr_4/1
  Gain/1 -> 整车动力学模型/1(需求车速 km/h)
  Pred_v3/1 -> Gain1/1
  Gain1/1 -> 整车动力学模型/2(需求车速 km/h1)

== system c221127_FCEV_SLMP_SQP/Subsystem4/VehModel_Pred+5 ==
  note: CarryOver
  Pred_v5 : Inport
  Pred_v1 : Inport  Port=2
  Enable : EnablePort
  Gain : Gain  Gain=3.6
  Gain1 : Gain  Gain=3.6
  Power bus : Subsystem
  主减及变速器模型 : Subsystem
  整车动力学模型 : Subsystem
  车轮模型 : Subsystem
  驱动电机模型 : Subsystem
  PredPwr_5 : Outport
  wires:
  主减及变速器模型/1(drive torque (Nm) speed (rad/s) brike torque (Nm) req'd at input side of final drive) -> 驱动电机模型/1(drive torque (Nm) speed (rad/s) brake torque (Nm) req'd at motor)
  驱动电机模型/1(drive power (kW) brake power (kW) req'd motor input power (电功率)) -> Power bus/1(drive power (kW) brake power (kW) req at power bus)
  整车动力学模型/1(需求驱动力N 目标车速m/s 需求制动力N) -> 车轮模型/1("tractive force, brake force and speed req'd of tire/road interface 需求驱动力N 目标车速m/s 需求制动力N")
  车轮模型/1(drive torque (Nm) speed (rad/s) brake torque (Nm) req'd from drivetrain into axle) -> 主减及变速器模型/1(drive torque (Nm) speed (rad/s) brake torque (Nm) req'd at output side of final drive)
  Pred_v5/1 -> Gain/1
  Power bus/1(drive power (kW)/brake power (kW) req from power sources) -> PredPwr_5/1
  Gain/1 -> 整车动力学模型/1(需求车速 km/h)
  Pred_v1/1 -> Gain1/1
  Gain1/1 -> 整车动力学模型/2(需求车速 km/h1)

== system c221127_FCEV_SLMP_SQP/Subsystem4/VehModel_Pred+6 ==
  note: CarryOver
  Pred_v6 : Inport
  Pred_v1 : Inport  Port=2
  Enable : EnablePort
  Gain : Gain  Gain=3.6
  Gain1 : Gain  Gain=3.6
  Power bus : Subsystem
  主减及变速器模型 : Subsystem
  整车动力学模型 : Subsystem
  车轮模型 : Subsystem
  驱动电机模型 : Subsystem
  PredPwr_6 : Outport
  wires:
  Gain/1 -> 整车动力学模型/1(需求车速 km/h)
  Power bus/1(drive power (kW)/brake power (kW) req from power sources) -> PredPwr_6/1
  Pred_v6/1 -> Gain/1
  车轮模型/1(drive torque (Nm) speed (rad/s) brake torque (Nm) req'd from drivetrain into axle) -> 主减及变速器模型/1(drive torque (Nm) speed (rad/s) brake torque (Nm) req'd at output side of final drive)
  整车动力学模型/1(需求驱动力N 目标车速m/s 需求制动力N) -> 车轮模型/1("tractive force, brake force and speed req'd of tire/road interface 需求驱动力N 目标车速m/s 需求制动力N")
  驱动电机模型/1(drive power (kW) brake power (kW) req'd motor input power (电功率)) -> Power bus/1(drive power (kW) brake power (kW) req at power bus)
  主减及变速器模型/1(drive torque (Nm) speed (rad/s) brike torque (Nm) req'd at input side of final drive) -> 驱动电机模型/1(drive torque (Nm) speed (rad/s) brake torque (Nm) req'd at motor)
  Pred_v1/1 -> Gain1/1
  Gain1/1 -> 整车动力学模型/2(需求车速 km/h1)

== system c221127_FCEV_SLMP_SQP/Subsystem4/VehModel_Pred+7 ==
  note: CarryOver
  Pred_v7 : Inport
  Pred_v1 : Inport  Port=2
  Enable : EnablePort
  Gain : Gain  Gain=3.6
  Gain1 : Gain  Gain=3.6
  Power bus : Subsystem
  主减及变速器模型 : Subsystem
  整车动力学模型 : Subsystem
  车轮模型 : Subsystem
  驱动电机模型 : Subsystem
  PredPwr_7 : Outport
  wires:
  Gain/1 -> 整车动力学模型/1(需求车速 km/h)
  Power bus/1(drive power (kW)/brake power (kW) req from power sources) -> PredPwr_7/1
  Pred_v7/1 -> Gain/1
  车轮模型/1(drive torque (Nm) speed (rad/s) brake torque (Nm) req'd from drivetrain into axle) -> 主减及变速器模型/1(drive torque (Nm) speed (rad/s) brake torque (Nm) req'd at output side of final drive)
  整车动力学模型/1(需求驱动力N 目标车速m/s 需求制动力N) -> 车轮模型/1("tractive force, brake force and speed req'd of tire/road interface 需求驱动力N 目标车速m/s 需求制动力N")
  驱动电机模型/1(drive power (kW) brake power (kW) req'd motor input power (电功率)) -> Power bus/1(drive power (kW) brake power (kW) req at power bus)
  主减及变速器模型/1(drive torque (Nm) speed (rad/s) brike torque (Nm) req'd at input side of final drive) -> 驱动电机模型/1(drive torque (Nm) speed (rad/s) brake torque (Nm) req'd at motor)
  Pred_v1/1 -> Gain1/1
  Gain1/1 -> 整车动力学模型/2(需求车速 km/h1)

== system c221127_FCEV_SLMP_SQP/Subsystem4/VehModel_Pred+8 ==
  note: CarryOver
  Pred_v8 : Inport
  Pred_v1 : Inport  Port=2
  Enable : EnablePort
  Gain : Gain  Gain=3.6
  Gain1 : Gain  Gain=3.6
  Power bus : Subsystem
  主减及变速器模型 : Subsystem
  整车动力学模型 : Subsystem
  车轮模型 : Subsystem
  驱动电机模型 : Subsystem
  PredPwr_8 : Outport
  wires:
  Gain/1 -> 整车动力学模型/1(需求车速 km/h)
  Power bus/1(drive power (kW)/brake power (kW) req from power sources) -> PredPwr_8/1
  Pred_v8/1 -> Gain/1
  车轮模型/1(drive torque (Nm) speed (rad/s) brake torque (Nm) req'd from drivetrain into axle) -> 主减及变速器模型/1(drive torque (Nm) speed (rad/s) brake torque (Nm) req'd at output side of final drive)
  整车动力学模型/1(需求驱动力N 目标车速m/s 需求制动力N) -> 车轮模型/1("tractive force, brake force and speed req'd of tire/road interface 需求驱动力N 目标车速m/s 需求制动力N")
  驱动电机模型/1(drive power (kW) brake power (kW) req'd motor input power (电功率)) -> Power bus/1(drive power (kW) brake power (kW) req at power bus)
  主减及变速器模型/1(drive torque (Nm) speed (rad/s) brike torque (Nm) req'd at input side of final drive) -> 驱动电机模型/1(drive torque (Nm) speed (rad/s) brake torque (Nm) req'd at motor)
  Pred_v1/1 -> Gain1/1
  Gain1/1 -> 整车动力学模型/2(需求车速 km/h1)

== system c221127_FCEV_SLMP_SQP/Subsystem4/VehModel_Pred+9 ==
  note: CarryOver
  Pred_v9 : Inport
  Pred_v1 : Inport  Port=2
  Enable : EnablePort
  Gain : Gain  Gain=3.6
  Gain1 : Gain  Gain=3.6
  Power bus : Subsystem
  主减及变速器模型 : Subsystem
  整车动力学模型 : Subsystem
  车轮模型 : Subsystem
  驱动电机模型 : Subsystem
  PredPwr_9 : Outport
  wires:
  Gain/1 -> 整车动力学模型/1(需求车速 km/h)
  Power bus/1(drive power (kW)/brake power (kW) req from power sources) -> PredPwr_9/1
  Pred_v9/1 -> Gain/1
  车轮模型/1(drive torque (Nm) speed (rad/s) brake torque (Nm) req'd from drivetrain into axle) -> 主减及变速器模型/1(drive torque (Nm) speed (rad/s) brake torque (Nm) req'd at output side of final drive)
  整车动力学模型/1(需求驱动力N 目标车速m/s 需求制动力N) -> 车轮模型/1("tractive force, brake force and speed req'd of tire/road interface 需求驱动力N 目标车速m/s 需求制动力N")
  驱动电机模型/1(drive power (kW) brake power (kW) req'd motor input power (电功率)) -> Power bus/1(drive power (kW) brake power (kW) req at power bus)
  主减及变速器模型/1(drive torque (Nm) speed (rad/s) brike torque (Nm) req'd at input side of final drive) -> 驱动电机模型/1(drive torque (Nm) speed (rad/s) brake torque (Nm) req'd at motor)
  Pred_v1/1 -> Gain1/1
  Gain1/1 -> 整车动力学模型/2(需求车速 km/h1)

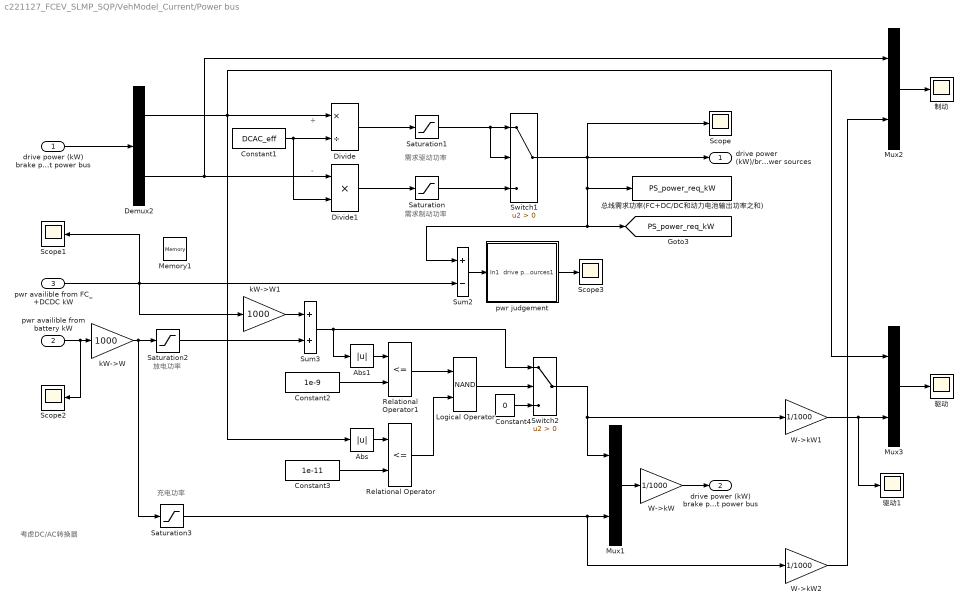
== system c221127_FCEV_SLMP_SQP/VehModel_Current/Power bus ==
  note: 充电功率
  note: 放电功率
  note: 考虑DC/AC转换器
  note: -
  note: +
  note: 需求制动功率
  note: 需求驱动功率
  drive power (kW) brake power (kW) req at power bus : Inport
  pwr availible from battery kW : Inport  Port=2
  pwr availible from FC_+DCDC kW : Inport  Port=3
  Abs : Abs  SaturateOnIntegerOverflow=off
  Abs1 : Abs  SaturateOnIntegerOverflow=off
  Constant1 : Constant  Value=DCAC_eff
  Constant2 : Constant  Value=1e-9
  Constant3 : Constant  Value=1e-11
  Constant4 : Constant  Value=0
  Demux2 : Demux  Outputs=2
  Divide : Product  Inputs=*/
  Divide1 : Product  Inputs=**
  Logical Operator : Logic  Operator=NAND  AllPortsSameDT=off  OutDataTypeStr=boolean
  Memory1 : Memory  InheritSampleTime=on
  Mux1 : Mux  Inputs=2
  Mux2 : Mux  Inputs=2
  Mux3 : Mux  Inputs=2
  Relational Operator : RelationalOperator  Operator=<=  OutDataTypeStr=boolean  InputSameDT=off
  Relational Operator1 : RelationalOperator  Operator=<=  OutDataTypeStr=boolean  InputSameDT=off
  Saturation : Saturate  UpperLimit=0  LowerLimit=-inf
  Saturation1 : Saturate  UpperLimit=inf  LowerLimit=0
  Saturation2 : Saturate  UpperLimit=inf  LowerLimit=0
  Saturation3 : Saturate  UpperLimit=0  LowerLimit=-inf
  Scope{,1..3} (4 alike) : Scope
  Sum2 : Sum  Inputs=+-
  Sum3 : Sum
  Switch1 : Switch  Criteria=u2 > Threshold  SaturateOnIntegerOverflow=off  InputSameDT=off
  Switch2 : Switch  Criteria=u2 > Threshold  SaturateOnIntegerOverflow=off  InputSameDT=off
  W->kW : Gain  Gain=1/1000
  W->kW1 : Gain  Gain=1/1000
  W->kW2 : Gain  Gain=1/1000
  kW->W : Gain  Gain=1000
  kW->W1 : Gain  Gain=1000
  pwr judgement : Subsystem
  制动 : Scope
  总线需求功率(FC+DC/DC和动力电池输出功率之和) : ToWorkspace  VariableName=PS_power_req_kW  SampleTime=-1
  驱动 : Scope
  驱动1 : Scope
  drive power (kW)/brake power (kW) req from power sources : Outport
  drive power (kW) brake power (kW) availableat power bus : Outport  Port=2
  tag scope: PS_power_req_kW=global
  wires:
  Abs1/1 -> Relational Operator1/1
  Constant2/1 -> Relational Operator1/2
  Constant1/1 -> Divide1/2, Divide/2
  Divide/1 -> Saturation1/1
  Divide1/1 -> Saturation/1
  drive power (kW) brake power (kW) req at power bus/1 -> Demux2/1
  Demux2/2 -> Mux2/1, Divide1/1
  Saturation1/1 -> Switch1/2, Switch1/1
  Switch1/1 -> drive power (kW)/brake power (kW) req from power sources/1, 总线需求功率(FC+DC/DC和动力电池输出功率之和)/1, Sum2/1, [PS_power_req_kW], Scope/1
  W->kW/1 -> drive power (kW) brake power (kW) availableat power bus/1
  Saturation/1 -> Switch1/3
  Mux2/1 -> 制动/1
  Mux3/1 -> 驱动/1
  W->kW1/1 -> 驱动1/1, Mux3/2
  W->kW2/1 -> Mux2/2
  Sum2/1 -> pwr judgement/1(In1)
  Saturation2/1 -> Sum3/2
  pwr availible from FC_+DCDC kW/1 -> kW->W1/1, Scope1/1, Sum2/2
  Sum3/1 -> Switch2/1, Abs1/1
  Relational Operator1/1 -> Logical Operator/1
  Abs/1 -> Relational Operator/1
  Constant3/1 -> Relational Operator/2
  Demux2/1 -> Mux3/1, Abs/1, Divide/1
  Relational Operator/1 -> Logical Operator/2
  Constant4/1 -> Switch2/3
  Logical Operator/1 -> Switch2/2
  Saturation3/1 -> W->kW2/1, Mux1/2
  Switch2/1 -> W->kW1/1, Mux1/1
  pwr availible from battery kW/1 -> Scope2/1, kW->W/1
  kW->W/1 -> Saturation3/1, Saturation2/1
  kW->W1/1 -> Sum3/1
  Mux1/1 -> W->kW/1
  pwr judgement/1(drive power (kW)/brake power (kW) req from power sources1) -> Scope3/1

== system c221127_FCEV_SLMP_SQP/VehModel_Current/主减及变速器模型 ==
  drive torque (Nm) speed (rad/s) brake torque (Nm) req'd at output side of final drive : Inport
  drive torque (Nm) brake torque (Nm) speed avail (rad/s) at input side of final drive : Inport  Port=2
  " Effect of inertia (Nm)1" : Subsystem
  Demux1 : Demux  Outputs=3
  Demux4 : Demux  Outputs=3
  Effect of inertia (Nm) : Subsystem
  Gain1 : Gain  Gain=1/Veh_final_drive_ratio
  Gain2 : Gain  Gain=1/Veh_final_drive_ratio
  Gain3 : Gain  Gain=Veh_final_drive_ratio  SaturateOnIntegerOverflow=on  OutDataTypeStr=Inherit: Same as input  ParamDataTypeStr=Inherit: Same as input
  Gain4 : Gain  Gain=1/Veh_final_drive_ratio  SaturateOnIntegerOverflow=on  OutDataTypeStr=Inherit: Same as input  ParamDataTypeStr=Inherit: Same as input
  Gain5 : Gain  Gain=Veh_final_drive_ratio  SaturateOnIntegerOverflow=on  OutDataTypeStr=Inherit: Same as input  ParamDataTypeStr=Inherit: Same as input
  Gain8 : Gain  Gain=Veh_final_drive_ratio  SaturateOnIntegerOverflow=on  OutDataTypeStr=Inherit: Same as input  ParamDataTypeStr=Inherit: Same as input
  Mux1 : Mux  Inputs=3
  Mux4 : Mux  Inputs=3
  Saturation : Saturate  UpperLimit=inf  LowerLimit=0
  Saturation1 : Saturate  UpperLimit=0  LowerLimit=-inf
  Saturation2 : Saturate  UpperLimit=inf  LowerLimit=0
  Scope : Scope
  Sum : Sum  Inputs=+++  InputSameDT=on  SaturateOnIntegerOverflow=on  OutDataTypeStr=Inherit: Same as first input
  Sum2 : Sum  Inputs=--+  InputSameDT=on  SaturateOnIntegerOverflow=on  OutDataTypeStr=Inherit: Same as first input
  Sum3 : Sum  Inputs=+++  InputSameDT=on  SaturateOnIntegerOverflow=on  OutDataTypeStr=Inherit: Same as first input
  Sum4 : Sum  Inputs=--+  InputSameDT=on  SaturateOnIntegerOverflow=on  OutDataTypeStr=Inherit: Same as first input
  loss (Nm) : Subsystem
  loss (Nm)1 : Subsystem
  主减速器需求制动转矩 : Scope
  主减速器需求转速 : Scope
  主减速器需求驱动转矩 : Scope
  drive torque (Nm) speed (rad/s) brike torque (Nm) req'd at input side of final drive : Outport  InitialOutput=0
  drive torque (Nm) brake torque (Nm) speed avail (rad/s) at output side of final drive : Outport  Port=2  InitialOutput=0
  wires:
  Demux4/2 -> Effect of inertia (Nm)/1(fd input speed (rad/s)), " Effect of inertia (Nm)1"/1(In1), Gain3/1
  Demux4/1 -> loss (Nm)/1("drive torque (Nm) "), Gain1/1
  Mux4/1 -> drive torque (Nm) speed (rad/s) brike torque (Nm) req'd at input side of final drive/1
  drive torque (Nm) speed (rad/s) brake torque (Nm) req'd at output side of final drive/1 -> Demux4/1
  Mux1/1 -> Scope/1, drive torque (Nm) brake torque (Nm) speed avail (rad/s) at output side of final drive/1
  drive torque (Nm) brake torque (Nm) speed avail (rad/s) at input side of final drive/1 -> Demux1/1
  Effect of inertia (Nm)/1(drag torque (Nm)) -> Sum2/2, Sum/2
  loss (Nm)/1(drag torque (Nm)) -> Sum2/1, Sum/1
  Gain1/1 -> Sum/3
  Sum/1 -> 主减速器需求驱动转矩/1, Mux4/1
  Gain3/1 -> 主减速器需求转速/1, Mux4/2
  " Effect of inertia (Nm)1"/1(Out1) -> Sum4/1, Sum3/2
  loss (Nm)1/1(drag torque (Nm)) -> Sum4/2, Sum3/3
  Demux4/3 -> Gain2/1, loss (Nm)1/1("drive torque (Nm) ")
  Gain2/1 -> Sum3/1
  Demux1/1 -> Sum2/3
  Demux1/2 -> Sum4/3
  Sum2/1 -> Gain8/1
  Gain8/1 -> Saturation/1
  Saturation/1 -> Mux1/1
  Sum4/1 -> Gain5/1
  Saturation1/1 -> Mux1/2
  Gain5/1 -> Saturation1/1
  Gain4/1 -> Saturation2/1
  Demux1/3 -> Gain4/1
  Saturation2/1 -> Mux1/3
  Sum3/1 -> 主减速器需求制动转矩/1, Mux4/3

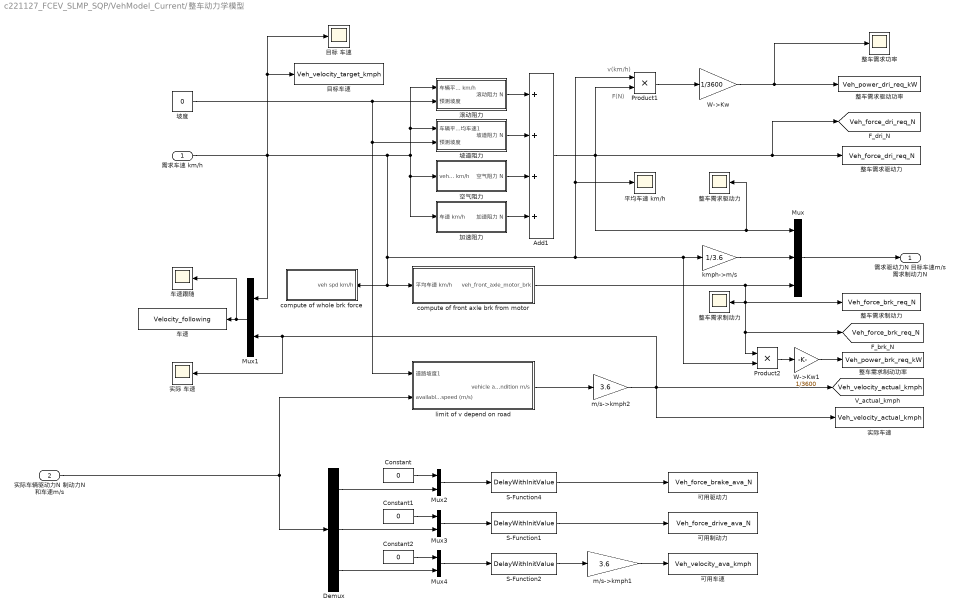
== system c221127_FCEV_SLMP_SQP/VehModel_Current/整车动力学模型 ==
  note: v(km/h)
  note: F(N)
  需求车速 km/h : Inport
  实际车辆驱动力N 制动力N 和车速m/s : Inport  Port=2
  "  整车需求制动力" : ToWorkspace  VariableName=Veh_force_brk_req_N  SaveFormat=Timeseries  SampleTime=-1
  "  整车需求制动功率" : ToWorkspace  VariableName=Veh_power_brk_req_kW  SampleTime=-1
  "  整车需求驱动力" : ToWorkspace  VariableName=Veh_force_dri_req_N  SaveFormat=Timeseries  SampleTime=-1
  "  整车需求驱动功率" : ToWorkspace  VariableName=Veh_power_dri_req_kW  SampleTime=-1
  "  目标车速" : ToWorkspace  VariableName=Veh_velocity_target_kmph  SaveFormat=Timeseries  SampleTime=-1
  "  车速" : ToWorkspace  VariableName=Velocity_following  SaveFormat=Timeseries  SampleTime=-1
  Add1 : Sum  Inputs=++++
  Constant : Constant  Value=0
  Constant1 : Constant  Value=0
  Constant2 : Constant  Value=0
  Demux : Demux  Outputs=3
  Mux : Mux  Inputs=3
  Mux{1..4} (4 alike) : Mux  Inputs=2
  Product1 : Product  RndMeth=Zero
  Product2 : Product  RndMeth=Zero
  S-Function1 : S-Function  FunctionName=DelayWithInitValue  SFunctionDeploymentMode=off  EnableBusSupport=off
  S-Function2 : S-Function  FunctionName=DelayWithInitValue  SFunctionDeploymentMode=off  EnableBusSupport=off
  S-Function4 : S-Function  FunctionName=DelayWithInitValue  SFunctionDeploymentMode=off  EnableBusSupport=off
  W->Kw : Gain  Gain=1/3600
  W->Kw1 : Gain  Gain=1/3600
  compute of front axle brk from motor : Subsystem
  compute of whole brk force : Subsystem
  kmph->m/s : Gain  Gain=1/3.6
  limit of v depend on road : Subsystem
  m/s->kmph1 : Gain  Gain=3.6
  m/s->kmph2 : Gain  Gain=3.6
  加速阻力 : Subsystem
  可用制动力 : ToWorkspace  VariableName=Veh_force_drive_ava_N  SaveFormat=Timeseries  SampleTime=-1
  可用车速 : ToWorkspace  VariableName=Veh_velocity_ava_kmph  SaveFormat=Timeseries  SampleTime=-1
  可用驱动力 : ToWorkspace  VariableName=Veh_force_brake_ava_N  SaveFormat=Timeseries  SampleTime=-1
  坡度 : Constant  Value=0
  坡道阻力 : Subsystem
  实际 车速 : Scope
  实际车速 : ToWorkspace  VariableName=Veh_velocity_actual_kmph  SaveFormat=Timeseries  SampleTime=-1
  平均车速 km/h : Scope
  整车需求制动力 : Scope
  整车需求功率 : Scope
  整车需求驱动力 : Scope
  滚动阻力 : Subsystem
  目标 车速 : Scope
  空气阻力 : Subsystem
  车速跟随 : Scope
  需求驱动力N 目标车速m/s 需求制动力N : Outport
  tag scope: Veh_force_brk_req_N=global, Veh_force_dri_req_N=global, Veh_velocity_actual_kmph=global
  wires:
  实际车辆驱动力N 制动力N 和车速m/s/1 -> limit of v depend on road/2(available drive force (N) brake force (N) and linear speed (m/s)), Demux/1
  滚动阻力/1(滚动阻力 N) -> Add1/1
  坡道阻力/1(坡道阻力 N) -> Add1/2
  空气阻力/1(空气阻力 N) -> Add1/3
  加速阻力/1(加速阻力 N) -> Add1/4
  Add1/1 -> 整车需求驱动力/1, Mux/1, [Veh_force_dri_req_N], "  整车需求驱动力"/1, Product1/2
  Mux/1 -> 需求驱动力N 目标车速m/s 需求制动力N/1
  Product1/1 -> W->Kw/1
  Demux/1 -> Mux2/2
  坡度/1 -> limit of v depend on road/1(道路坡度1), 坡道阻力/2(预测坡度), 滚动阻力/2(预测坡度)
  W->Kw/1 -> "  整车需求驱动功率"/1, 整车需求功率/1
  kmph->m/s/1 -> Mux/2
  limit of v depend on road/1(vehicle achievable consider of the road condition m/s) -> m/s->kmph2/1
  m/s->kmph2/1 -> 实际车速/1, Mux1/2, 实际 车速/1, [Veh_velocity_actual_kmph]
  需求车速 km/h/1 -> 目标 车速/1, "  目标车速"/1, compute of front axle brk from motor/1(平均车速 km/h), compute of whole brk force/1(veh spd km/h), Product2/2, kmph->m/s/1, 平均车速 km/h/1, Product1/1, 加速阻力/1(车速 km/h), 空气阻力/1(veh_spd km/h), 滚动阻力/1(车辆平均车速 km/h), 坡道阻力/1(车辆平均车速1), Mux1/1
  m/s->kmph1/1 -> 可用车速/1
  compute of front axle brk from motor/1(veh_front_axle_motor_brk) -> Mux/3, 整车需求制动力/1, "  整车需求制动力"/1, [Veh_force_brk_req_N], Product2/1
  Product2/1 -> W->Kw1/1
  W->Kw1/1 -> "  整车需求制动功率"/1
  Demux/3 -> Mux4/2
  Demux/2 -> Mux3/2
  Mux1/1 -> "  车速"/1, 车速跟随/1
  Constant/1 -> Mux2/1
  Mux2/1 -> S-Function4/1
  S-Function4/1 -> 可用驱动力/1
  Mux3/1 -> S-Function1/1
  Constant1/1 -> Mux3/1
  Constant2/1 -> Mux4/1
  Mux4/1 -> S-Function2/1
  S-Function1/1 -> 可用制动力/1
  S-Function2/1 -> m/s->kmph1/1
